simulink model "tracking_control"  (Simulink 8.6)
settings: Solver=ode45  StartTime=0.0  StopTime=500  MaxStep=0.02  RelTol=1e-3
values from neighbouring files (symbols this model uses):
  D = [dxd+bb1;dyd+bb2]    [alfuv.m]    (also in constant.m = diag([d11,d22,d33]))
  K01 = diag([1,1,1])    [constant.m]
  M = diag([m11,m22,m33])    [constant.m]
libraries: simulink x2
settings Model: Creator=Administrator  LastModifiedBy=Administrator
settings DebuggingCC: AlgebraicLoopMsg=none  SolverPrmCheckMsg=none  FcnCallInpInsideContextMsg=EnableAllAsWarning
settings GRTTargetCC: CombineOutputUpdateFcns=on  GRTInterface=off

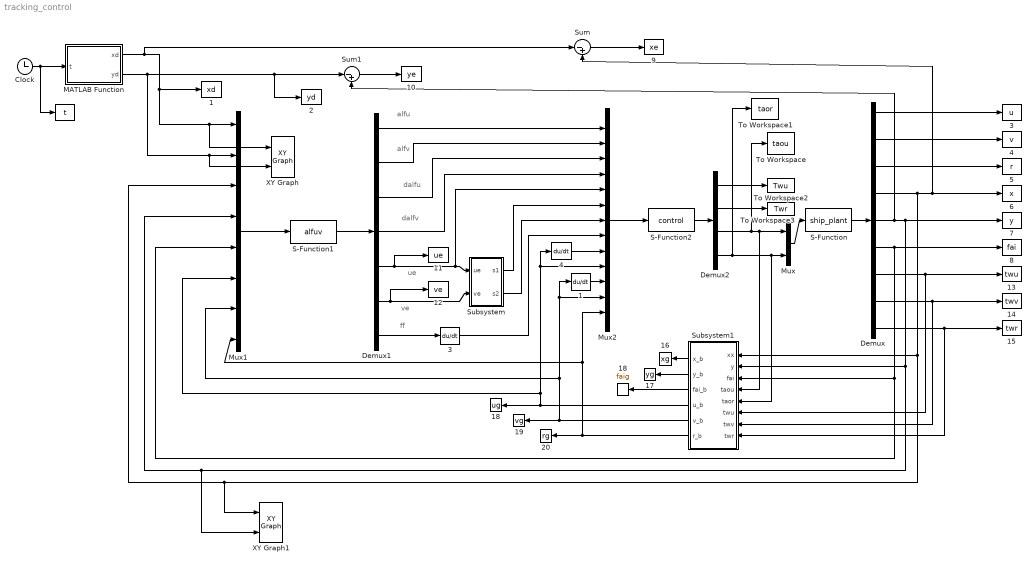
== system tracking_control ==
  note: alfu
  note: alfv
  note: dalfu
  note: dalfv
  note: ue
  note: ve
  note: ff
  " " : ToWorkspace  VariableName=t  SampleTime=-1
  "   1" : Derivative
  "   3" : Derivative
  "   4" : Derivative
  " 1" : ToWorkspace  VariableName=xd  SampleTime=-1
  " 10" : ToWorkspace  VariableName=ye  SampleTime=-1
  " 11" : ToWorkspace  VariableName=ue  SampleTime=-1
  " 12" : ToWorkspace  VariableName=ve  SampleTime=-1
  " 13" : ToWorkspace  VariableName=twu  SampleTime=-1
  " 14" : ToWorkspace  VariableName=twv  SampleTime=-1
  " 15" : ToWorkspace  VariableName=twr  SampleTime=-1
  " 16" : ToWorkspace  VariableName=xg  SampleTime=-1
  " 17" : ToWorkspace  VariableName=yg  SampleTime=-1
  " 18" : ToWorkspace  VariableName=ug  SampleTime=-1
  " 19" : ToWorkspace  VariableName=vg  SampleTime=-1
  " 2" : ToWorkspace  VariableName=yd  SampleTime=-1
  " 20" : ToWorkspace  VariableName=rg  SampleTime=-1
  " 3" : ToWorkspace  VariableName=u  SampleTime=-1
  " 4" : ToWorkspace  VariableName=v  SampleTime=-1
  " 5" : ToWorkspace  VariableName=r  SampleTime=-1
  " 6" : ToWorkspace  VariableName=x  SampleTime=-1
  " 7" : ToWorkspace  VariableName=y  SampleTime=-1
  " 8" : ToWorkspace  VariableName=fai  SampleTime=-1
  " 9" : ToWorkspace  VariableName=xe  SampleTime=-1
  18 : ToWorkspace  VariableName=faig  SampleTime=-1
  Clock : Clock
  Demux : Demux  Outputs=9
  Demux1 : Demux  Outputs=7
  Demux2 : Demux
  MATLAB Function : MATLAB Function  TreatAsAtomicUnit=on
  Mux : Mux  Inputs=2
  Mux1 : Mux  Inputs=8
  Mux2 : Mux  Inputs=13
  S-Function : S-Function  FunctionName=ship_plant  SFunctionDeploymentMode=off  EnableBusSupport=off
  S-Function1 : S-Function  FunctionName=alfuv  SFunctionDeploymentMode=off  EnableBusSupport=off
  S-Function2 : S-Function  FunctionName=control  SFunctionDeploymentMode=off  EnableBusSupport=off
  Subsystem : Subsystem
  Subsystem1 : Subsystem
  Sum : Sum  Inputs=|-+
  Sum1 : Sum  Inputs=|-+
  To Workspace : ToWorkspace  VariableName=taou  SampleTime=-1
  To Workspace1 : ToWorkspace  VariableName=taor  SampleTime=-1
  To Workspace2 : ToWorkspace  VariableName=Twu  SampleTime=-1
  To Workspace3 : ToWorkspace  VariableName=Twr  SampleTime=-1
  XY Graph : simulink/Sinks/XY Graph  xmin=-500  xmax=500  ymin=-500  ymax=500  st=-1
  XY Graph1 : simulink/Sinks/XY Graph  xmin=-500  xmax=500  ymin=-500  ymax=500  st=-1
  wires:
  Clock/1 -> MATLAB Function/1(t), " "/1
  MATLAB Function/2(yd) -> Sum1/1, " 2"/1, Mux1/2, XY Graph/2
  MATLAB Function/1(xd) -> Sum/1, " 1"/1, Mux1/1, XY Graph/1
  S-Function/1 -> Demux/1
  Demux/1 -> " 3"/1
  Demux/2 -> " 4"/1
  Demux/3 -> " 5"/1
  Demux/4 -> " 6"/1, Sum/2, Subsystem1/1(xx), Mux1/3, XY Graph1/1
  Demux/5 -> " 7"/1, Subsystem1/2(y), Mux1/4, XY Graph1/2, Sum1/2
  Demux/6 -> " 8"/1, Mux1/5, Subsystem1/3(fai)
  Mux/1 -> S-Function/1
  Mux1/1 -> S-Function1/1
  S-Function1/1 -> Demux1/1
  Demux1/1 -> Mux2/1
  S-Function2/1 -> Demux2/1
  Demux1/2 -> Mux2/2
  Demux1/3 -> Mux2/3
  Demux1/4 -> Mux2/4
  Demux1/5 -> Mux2/5, Subsystem/1(ue), " 11"/1
  Demux1/6 -> Subsystem/2(ve), " 12"/1
  Demux1/7 -> "   3"/1
  Mux2/1 -> S-Function2/1
  Subsystem/1(s1) -> Mux2/6
  Subsystem/2(s2) -> Mux2/7
  "   3"/1 -> Mux2/8
  "   4"/1 -> Mux2/9
  "   1"/1 -> Mux2/11
  Sum/1 -> " 9"/1
  Sum1/1 -> " 10"/1
  Demux2/3 -> To Workspace/1, Mux/1, Subsystem1/4(taou)
  Demux2/4 -> To Workspace1/1, Mux/2, Subsystem1/5(taor)
  Demux2/2 -> To Workspace3/1
  Demux2/1 -> To Workspace2/1
  Demux/7 -> " 13"/1, Subsystem1/6(twu)
  Demux/8 -> " 14"/1, Subsystem1/7(twv)
  Demux/9 -> " 15"/1, Subsystem1/8(twr)
  Subsystem1/1(x_b) -> " 16"/1
  Subsystem1/2(y_b) -> " 17"/1
  Subsystem1/3(fai_b) -> 18/1
  Subsystem1/4(u_b) -> " 18"/1, "   4"/1, Mux2/10, Mux1/6
  Subsystem1/5(v_b) -> " 19"/1, "   1"/1, Mux2/12, Mux1/7
  Subsystem1/6(r_b) -> " 20"/1, Mux2/13, Mux1/8

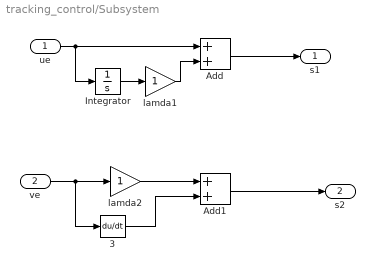
== system tracking_control/Subsystem ==
  ue : Inport
  ve : Inport  Port=2
  "   3" : Derivative
  Add : Sum
  Add1 : Sum
  Integrator : Integrator
  lamda1 : Gain
  lamda2 : Gain
  s1 : Outport
  s2 : Outport  Port=2
  wires:
  ue/1 -> Add/1, Integrator/1
  Integrator/1 -> lamda1/1
  lamda1/1 -> Add/2
  Add/1 -> s1/1
  ve/1 -> lamda2/1, "   3"/1
  lamda2/1 -> Add1/1
  "   3"/1 -> Add1/2
  Add1/1 -> s2/1

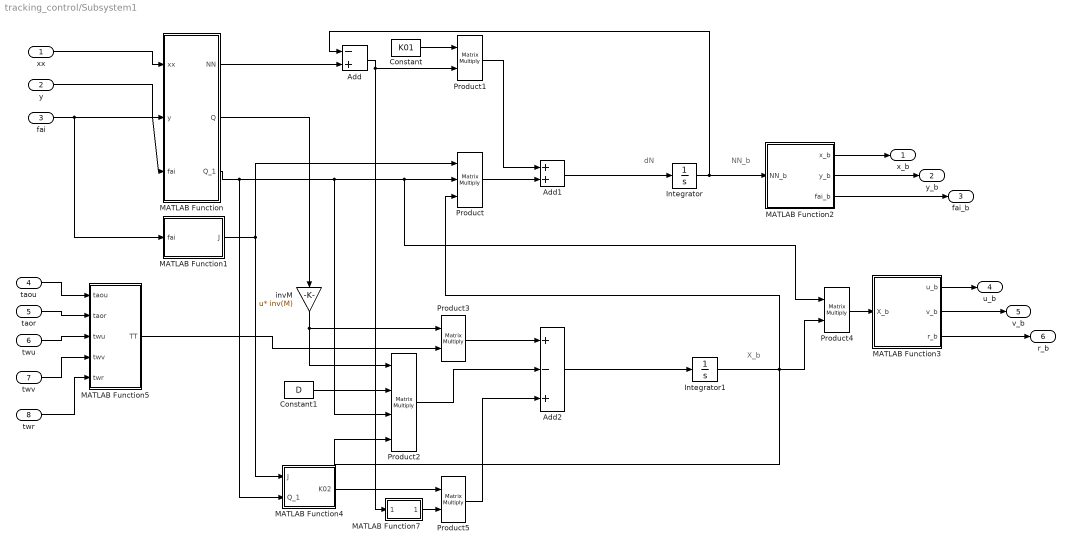
== system tracking_control/Subsystem1 ==
  note: X_b
  note: NN_b
  note: dN
  xx : Inport
  y : Inport  Port=2
  fai : Inport  Port=3
  taou : Inport  Port=4
  taor : Inport  Port=5
  twu : Inport  Port=6
  twv : Inport  Port=7
  twr : Inport  Port=8
  Add : Sum  Inputs=-+
  Add1 : Sum
  Add2 : Sum  Inputs=+-+
  Constant : Constant  Value=K01
  Constant1 : Constant  Value=D
  Integrator : Integrator
  Integrator1 : Integrator  InitialCondition=[0;0;0.5]
  MATLAB Function : MATLAB Function  TreatAsAtomicUnit=on
  MATLAB Function1 : MATLAB Function  TreatAsAtomicUnit=on
  MATLAB Function2 : MATLAB Function  TreatAsAtomicUnit=on
  MATLAB Function3 : MATLAB Function  TreatAsAtomicUnit=on
  MATLAB Function4 : MATLAB Function  TreatAsAtomicUnit=on
  MATLAB Function5 : MATLAB Function  TreatAsAtomicUnit=on
  MATLAB Function7 : MATLAB Function  TreatAsAtomicUnit=on
  Product : Product  Inputs=3  Multiplication=Matrix(*)  RndMeth=Zero
  Product{1,3..5} (4 alike) : Product  Multiplication=Matrix(*)  RndMeth=Zero
  Product2 : Product  Inputs=4  Multiplication=Matrix(*)  RndMeth=Zero
  invM : Gain  Gain=inv(M)  Multiplication=Matrix(u*K)
  x_b : Outport
  y_b : Outport  Port=2
  fai_b : Outport  Port=3
  u_b : Outport  Port=4
  v_b : Outport  Port=5
  r_b : Outport  Port=6
  wires:
  Product4/1 -> MATLAB Function3/1(X_b)
  MATLAB Function3/3(r_b) -> r_b/1
  MATLAB Function3/2(v_b) -> v_b/1
  MATLAB Function3/1(u_b) -> u_b/1
  MATLAB Function2/3(fai_b) -> fai_b/1
  MATLAB Function2/2(y_b) -> y_b/1
  MATLAB Function2/1(x_b) -> x_b/1
  Add2/1 -> Integrator1/1
  Product2/1 -> Add2/2
  Product3/1 -> Add2/1
  Constant1/1 -> Product2/2
  invM/1 -> Product2/1, Product3/1
  MATLAB Function/2(Q) -> invM/1
  Constant/1 -> Product1/1
  Add/1 -> MATLAB Function7/1(ETA), Product1/2
  MATLAB Function/1(NN) -> Add/2
  MATLAB Function1/1(J) -> Product/1, MATLAB Function4/1(J)
  MATLAB Function/3(Q_1) -> Product2/3, Product/2, Product4/1, MATLAB Function4/2(Q_1)
  Product1/1 -> Add1/1
  Integrator/1 -> Add/1, MATLAB Function2/1(NN_b)
  Product/1 -> Add1/2
  Integrator1/1 -> Product/3, Product2/4, Product4/2
  Add1/1 -> Integrator/1
  fai/1 -> MATLAB Function/3(fai), MATLAB Function1/1(fai)
  y/1 -> MATLAB Function/2(y)
  xx/1 -> MATLAB Function/1(xx)
  MATLAB Function4/1(K02) -> Product5/1
  Product5/1 -> Add2/3
  taou/1 -> MATLAB Function5/1(taou)
  taor/1 -> MATLAB Function5/2(taor)
  twu/1 -> MATLAB Function5/3(twu)
  twv/1 -> MATLAB Function5/4(twv)
  twr/1 -> MATLAB Function5/5(twr)
  MATLAB Function5/1(TT) -> Product3/2
  MATLAB Function7/1(YY2) -> Product5/2

== matlab function Subsystem1/MATLAB Function ==
  data: xx input double; y input double; fai input double; NN output double; Q output double; Q_1 output double
function [NN,Q,Q_1] = fcn(xx,y,fai)
%#codegen
m11=1.2*10^5;m22=1.779*10^5;m33=6.36*10^7;
d11=2.15*10^4;d22=1.47*10^5;d33=8.02*10^6;
NN=[xx;y;fai];
% TAO=[taou;0;taor];
alfa=m22/m11;
beta=m11/m33;
gama=m22/m33;
f=xx*sin(fai)-y*cos(fai);
h=xx*cos(fai)+y*sin(fai);
Q =[cos(fai) -alfa*sin(fai) 0;sin(fai) alfa*cos(fai) 0;f*beta h*gama 1];
Q_1=inv(Q);

== matlab function MATLAB Function ==
  data: t input double; xd output double; yd output double
function [xd,yd]= fcn(t)
%#codegen
% xd=200*sin(0.02*t+pi/4);
% yd=200*cos(0.02*t+pi/4);
% xd=200*sin(0.02*t);
% yd=200*cos(0.02*t);
xd=300*sin(0.03*t);
yd=300*cos(0.03*t);

== matlab function Subsystem1/MATLAB Function1 ==
  data: fai input double; J output double
function J = fcn(fai)
%#codegen

J=[cos(fai) -sin(fai) 0;
    sin(fai) cos(fai) 0;
    0 0 1];

== matlab function Subsystem1/MATLAB Function2 ==
  data: NN_b input double; x_b output double; y_b output double; fai_b output double
function [x_b,y_b,fai_b] = fcn(NN_b)
%#codegen

x_b=[1 0 0]*NN_b;
y_b=[0 1 0]*NN_b;
fai_b=[0 0 1]*NN_b;

== matlab function Subsystem1/MATLAB Function3 ==
  data: X_b input double; u_b output double; v_b output double; r_b output double
function [u_b,v_b,r_b] = fcn(X_b)
%#codegen

u_b=[1 0 0]*X_b;
v_b=[0 1 0]*X_b;
r_b=[0 0 1]*X_b;

== matlab function Subsystem1/MATLAB Function4 ==
  data: J input double; K02 output double; Q_1 input double
function K02= fcn(J,Q_1)
%#codegen

K02=(J*Q_1)';

== matlab function Subsystem1/MATLAB Function5 ==
  data: taou input double; taor input double; twu input double; twv input double; twr input double; TT output double
function TT = fcn(taou,taor,twu,twv,twr)
%#codegen
TAO=[taou;0;taor];
TW=[twu;twv;twr];
TT=TAO+TW;

== matlab function Subsystem1/MATLAB Function7 ==
  data: ETA input double; YY2 output double
function YY2 = fcn(ETA)
%#codegen
x1=[1 0 0]*ETA;
x2=[0 1 0]*ETA;
x3=[0 0 1]*ETA;
y1=(abs(x1))^(1/2)*sign(x1);
y2=(abs(x2))^(1/2)*sign(x2);
y3=(abs(x3))^(1/2)*sign(x3);
YY2 = [y1;y2;y3];
